simulink model "UAV_TAILSITTER_MODEL"  (R2023a)
settings: Solver=FixedStepAuto  StartTime=0.0  StopTime=60  FixedStep=0.001  RelTol=1e-3
libraries: vrlib x1
settings Model: Creator=kiqMC  LastModifiedBy=kiqMC
settings OptimizationCC: ReuseModelBlockBuffer=off

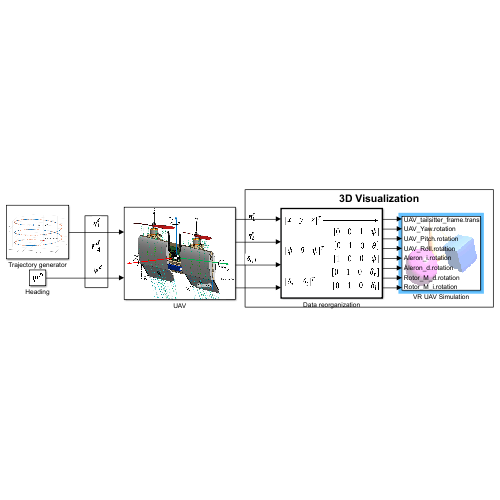
[thumbnail: Simulink's stored preview of the top-level diagram]
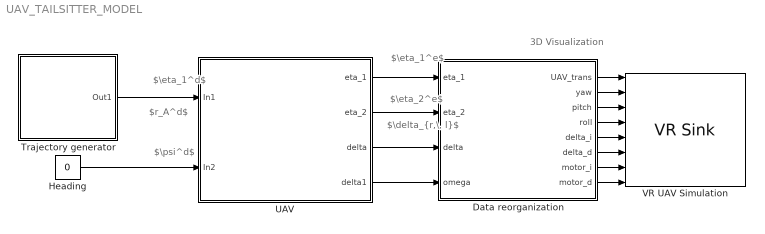
== system UAV_TAILSITTER_MODEL ==
  note: 3D Visualization
  note: $r_A^d$
  note: $\delta_{r,\, l}$
  note: $\eta_1^e$
  note: $\psi^d$
  note: $\eta_1^d$
  note: $\eta_2^e$
  Data reorganization : MATLAB Function  TreatAsAtomicUnit=on
  Heading : Constant  Value=0
      mask Display: image('C:\Users\kiqMC\Dropbox\Proyecto de Tesis MAC\psi_des.png'); % Use "Edit Image" on toolstrip to change.
  Trajectory generator : Subsystem
      mask Display: image('C:\Users\kiqMC\Dropbox\Proyecto de Tesis MAC\trajectoria.png'); % Use "Edit Image" on toolstrip to change.
  UAV : Subsystem
      mask Display: image('C:\Users\kiqMC\Dropbox\Tesis Enrique Mar\Modelo\Simulador UAV\Imágenes\UAV Fuerzas pares.png'); % Use "Edit Image" on toolstrip to change.
  VR UAV Simulation : vrlib/VR Sink  InstantiateOnLoad=on  SampleTime=0.05  ViewEnable=on  RemoteChange=off  RemoteView=off  FieldsWritten=UAV_tailsitter_frame.translation.3.1.1.double#UAV_Yaw.rotation.4.1.1.double#UAV_Pitch.rotation.4.1.1.double#UAV_Roll.rotation.4.1.1.double#Aleron_i.rotation.4.1.1.double#Aleron_d.rotation.4.1.1.double#Rotor_M_d.rotation.4.1.1.double#Rotor_M_i.rotation.4.1.1.double  WorldFileName=C:\Users\kiqMC\Dropbox\Proyecto de Tesis MAC\Diseño CAD drone\Tailsitter 0.3\UAV tailsitter ENSAMBLE MATLAB\uav world motors.wrl  AutoView=off  VideoDimensions=[]  AllowVariableSize=off
  wires:
  Trajectory generator/1(Out1) -> UAV/1(In1)
  UAV/1(eta_1) -> Data reorganization/1(eta_1)
  UAV/2(eta_2) -> Data reorganization/2(eta_2)
  UAV/3(delta) -> Data reorganization/3(delta)
  Heading/1 -> UAV/2(In2)
  UAV/4(delta1) -> Data reorganization/4(omega)
  Data reorganization/1(UAV_trans) -> VR UAV Simulation/1
  Data reorganization/2(yaw) -> VR UAV Simulation/2
  Data reorganization/3(pitch) -> VR UAV Simulation/3
  Data reorganization/4(roll) -> VR UAV Simulation/4
  Data reorganization/5(delta_i) -> VR UAV Simulation/5
  Data reorganization/6(delta_d) -> VR UAV Simulation/6
  Data reorganization/7(motor_i) -> VR UAV Simulation/7
  Data reorganization/8(motor_d) -> VR UAV Simulation/8

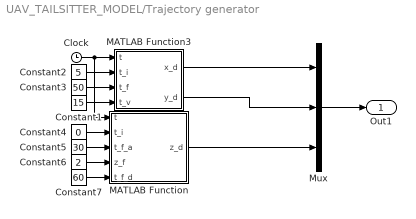
== system UAV_TAILSITTER_MODEL/Trajectory generator ==
  Clock : Clock
  Constant1 : Constant  Value=15
  Constant2 : Constant  Value=5
  Constant3 : Constant  Value=50
  Constant4 : Constant  Value=0
  Constant5 : Constant  Value=30
  Constant6 : Constant  Value=2
  Constant7 : Constant  Value=60
  MATLAB Function : MATLAB Function  TreatAsAtomicUnit=on
  MATLAB Function3 : MATLAB Function  TreatAsAtomicUnit=on
  Mux : Mux  Inputs=3
  Out1 : Outport
  wires:
  MATLAB Function/1(z_d) -> Mux/3
  Constant5/1 -> MATLAB Function/3(t_f_a)
  Constant7/1 -> MATLAB Function/5(t_f_d)
  Constant4/1 -> MATLAB Function/2(t_i)
  Clock/1 -> MATLAB Function/1(t), MATLAB Function3/1(t)
  Constant1/1 -> MATLAB Function3/4(t_v)
  MATLAB Function3/2(y_d) -> Mux/2
  Constant2/1 -> MATLAB Function3/2(t_i)
  MATLAB Function3/1(x_d) -> Mux/1
  Constant3/1 -> MATLAB Function3/3(t_f)
  Constant6/1 -> MATLAB Function/4(z_f)
  Mux/1 -> Out1/1

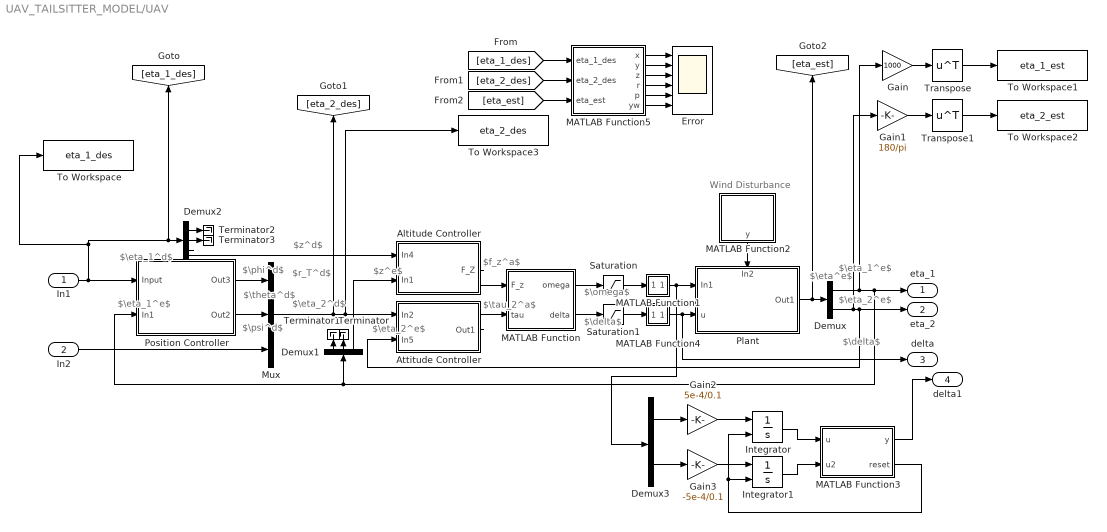
== system UAV_TAILSITTER_MODEL/UAV ==
  note: Wind Disturbance
  note: $\eta^e$
  note: $\eta_2^e$
  note: $\eta_1^e$
  note: $r_T^d$
  note: $z^d$
  note: $z^e$
  note: $\eta_1^d$
  note: $\eta_1^e$
  note: $\eta_2^d$
  note: $\tau_2^a$
  note: $\eta_2^e$
  note: $\omega$
  note: $f_z^a$
  note: $\delta$
  note: $\psi^d$
  note: $\phi^d$
  note: $\theta^d$
  note: $\delta$
  In1 : Inport
  In2 : Inport  Port=2
  Altitude Controller : Subsystem
      mask Display: image('C:\Users\kiqMC\Dropbox\Tesis Enrique Mar\Modelo\Simulador UAV\Imágenes\UAV altitud.png'); % Use "Edit Image" on toolstrip to change.
  Attitude Controller : Subsystem
      mask Display: image('C:\Users\kiqMC\Dropbox\Tesis Enrique Mar\Modelo\Simulador UAV\Imágenes\attitude.png'); % Use "Edit Image" on toolstrip to change.
  Demux : Demux  Outputs=2
  Demux1 : Demux  Outputs=3
  Demux2 : Demux  Outputs=3
  Demux3 : Demux  Outputs=2
  Error : Scope  NumInputPorts=6
  Gain : Gain  Gain=1000
  Gain1 : Gain  Gain=180/pi
  Gain2 : Gain  Gain=5e-4/0.1
  Gain3 : Gain  Gain=-5e-4/0.1
  Integrator : Integrator  ExternalReset=rising  InitialCondition=-180
  Integrator1 : Integrator  ExternalReset=rising  InitialCondition=180
  MATLAB Function : MATLAB Function  TreatAsAtomicUnit=on
  MATLAB Function1 : MATLAB Function  TreatAsAtomicUnit=on
  MATLAB Function2 : MATLAB Function  TreatAsAtomicUnit=on
  MATLAB Function3 : MATLAB Function  TreatAsAtomicUnit=on
  MATLAB Function4 : MATLAB Function  TreatAsAtomicUnit=on
  MATLAB Function5 : MATLAB Function  TreatAsAtomicUnit=on
  Mux : Mux  Inputs=3
  Plant : Subsystem
      settings: PortSchema="{\"entries\":[{\"content\":{\"sides\":[{\"content\":{\"connectorIds\":[\"In1\",\"In2\"]},\"type\":\"ConnectorPlacement.EquallySpacedRectSide\",\"uuid\":\"7724979e-19ed-4aea-9b0c-b20c5897cfe4\"},{\"content\":{\"connectorIds\":[\"Out1\"],\"side\":\"RIGHT\"},\"type\":\"ConnectorPlacement.EquallySpacedRectSide\",\"uuid\":\"79b46cc9-feaa-4989-867f-3ea67bf432a4\"},{\"content\":{\"connectorIds\":[\"In3\"],\"side\":\"TOP\"},\"type\":\"ConnectorPlacement.EquallySpacedRectSide\",\"uuid\":\"47fc0c27-c95e-4a7c-a970-96a958cf5736\"}]},\"type\":\"ConnectorPlacement.EquallySpacedConnector\",\"uuid\":\"a2521353-5775-4b64-ae3f-968c3914afab\"}],\"packageUris\":[\"http://schema.mathworks.com/mf0/Connector/R2020b\"],\"version\":\"1.0\"}"
      mask Display: image('C:\Users\kiqMC\Dropbox\Tesis Enrique Mar\Modelo\Simulador UAV\Imágenes\1.png'); % Use "Edit Image" on toolstrip to change.
  Position Controller : Subsystem
      mask Display: image('C:\Users\kiqMC\Dropbox\Tesis Enrique Mar\Modelo\Simulador UAV\Imágenes\position.png'); % Use "Edit Image" on toolstrip to change.
  Saturation : Saturate  UpperLimit=11000  LowerLimit=9600
  Saturation1 : Saturate  UpperLimit=10*pi/180  LowerLimit=-10*pi/180
  Terminator{,1..3} (4 alike) : Terminator
  To Workspace : ToWorkspace  VariableName=eta_1_des  SampleTime=-1
      settings: Save2DSignal=2-D array (concatenate along first dimension)
  To Workspace1 : ToWorkspace  VariableName=eta_1_est  SampleTime=-1
      settings: Save2DSignal=2-D array (concatenate along first dimension)
  To Workspace2 : ToWorkspace  VariableName=eta_2_est  SampleTime=-1
      settings: Save2DSignal=2-D array (concatenate along first dimension)
  To Workspace3 : ToWorkspace  VariableName=eta_2_des  SampleTime=-1
      settings: Save2DSignal=2-D array (concatenate along first dimension)
  Transpose : Math  Operator=transpose
  Transpose1 : Math  Operator=transpose
  eta_1 : Outport
  eta_2 : Outport  Port=2
  delta : Outport  Port=3
  delta1 : Outport  Port=4
  wires:
  [eta_1_des] -> MATLAB Function5/1(eta_1_des)
  Position Controller/1(Out3) -> Mux/1
  [eta_2_des] -> MATLAB Function5/2(eta_2_des)
  MATLAB Function5/5(p) -> Error/5
  MATLAB Function/1(omega) -> Saturation/1
  Demux2/3 -> Altitude Controller/1(In4)
  MATLAB Function1/1(y) -> Demux3/1, Plant/1(In1)
  Saturation/1 -> MATLAB Function1/1(u)
  Saturation1/1 -> MATLAB Function4/1(u)
  Demux/1 -> Gain/1, eta_1/1, Position Controller/2(In1), Demux1/1
  [eta_est] -> MATLAB Function5/3(eta_est)
  Plant/1(Out1) -> [eta_est], Demux/1
  MATLAB Function4/1(y) -> delta/1, Plant/2(u)
  Position Controller/2(Out2) -> Mux/2
  Demux/2 -> eta_2/1, Attitude Controller/2(In5), Gain1/1
  Demux2/2 -> Terminator3/1
  MATLAB Function5/3(z) -> Error/3
  Mux/1 -> [eta_2_des], To Workspace3/1, Attitude Controller/1(In2)
  Attitude Controller/1(Out1) -> MATLAB Function/2(tau)
  MATLAB Function5/4(r) -> Error/4
  Demux2/1 -> Terminator2/1
  Demux1/2 -> Terminator/1
  MATLAB Function/2(delta) -> Saturation1/1
  Demux1/1 -> Terminator1/1
  Demux1/3 -> Altitude Controller/2(In1)
  MATLAB Function5/2(y) -> Error/2
  MATLAB Function5/1(x) -> Error/1
  MATLAB Function5/6(yw) -> Error/6
  In1/1 -> Position Controller/1(Input), To Workspace/1, [eta_1_des], Demux2/1
  In2/1 -> Mux/3
  Altitude Controller/1(F_Z) -> MATLAB Function/1(F_z)
  MATLAB Function2/1(y) -> Plant/3(In2)
  Transpose/1 -> To Workspace1/1
  Transpose1/1 -> To Workspace2/1
  Gain/1 -> Transpose/1
  Gain1/1 -> Transpose1/1
  Integrator/1 -> MATLAB Function3/1(u)
  Gain2/1 -> Integrator/1
  MATLAB Function3/1(y) -> delta1/1
  MATLAB Function3/2(reset) -> Integrator/2, Integrator1/2
  Integrator1/1 -> MATLAB Function3/2(u2)
  Gain3/1 -> Integrator1/1
  Demux3/1 -> Gain2/1
  Demux3/2 -> Gain3/1

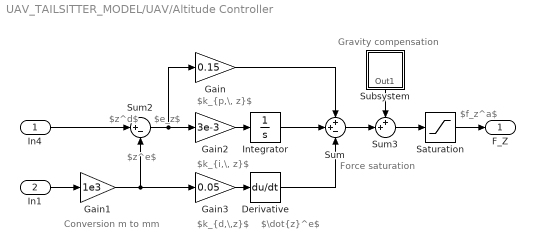
== system UAV_TAILSITTER_MODEL/UAV/Altitude Controller ==
  note: Conversion
      | m to mm
  note: $\dot{z}^e$
  note: $e_z$
  note: $f_z^a$
  note: Force saturation
  note: Gravity compensation
  note: $z^e$
  note: $z^d$
  note: $k_{p,\, z}$
  note: $k_{i,\, z}$
  note: $k_{d,\,z}$
  In4 : Inport
  In1 : Inport  Port=2
  Derivative : Derivative
  Gain : Gain  Gain=0.15
  Gain1 : Gain  Gain=1e3
  Gain2 : Gain  Gain=3e-3
  Gain3 : Gain  Gain=0.05
  Integrator : Integrator
  Saturation : Saturate  UpperLimit=13.791  LowerLimit=8.791
  Subsystem : Subsystem
      mask Display: image('C:\Users\kiqMC\Dropbox\Tesis Enrique Mar\Modelo\Simulador UAV\Imágenes\gravity.png'); % Use "Edit Image" on toolstrip to change.
  Sum : Sum  Inputs=++-
  Sum2 : Sum  Inputs=|+-
  Sum3 : Sum  Inputs=++|
  F_Z : Outport
  wires:
  Gain1/1 -> Sum2/2, Gain3/1
  In4/1 -> Sum2/1
  In1/1 -> Gain1/1
  Gain3/1 -> Derivative/1
  Gain2/1 -> Integrator/1
  Sum2/1 -> Gain2/1, Gain/1
  Integrator/1 -> Sum/2
  Gain/1 -> Sum/1
  Derivative/1 -> Sum/3
  Saturation/1 -> F_Z/1
  Sum/1 -> Sum3/2
  Sum3/1 -> Saturation/1
  Subsystem/1(Out1) -> Sum3/1

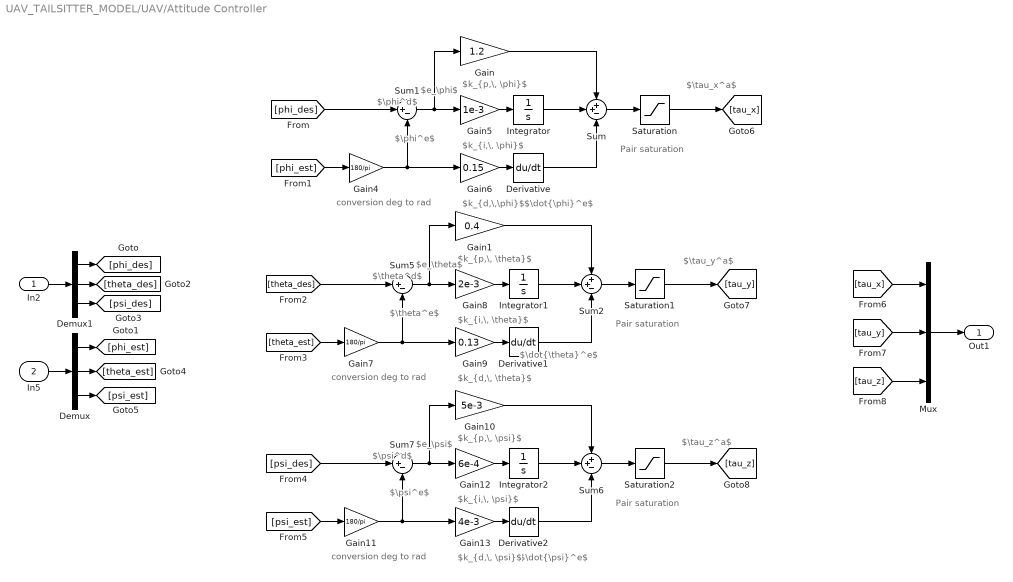
== system UAV_TAILSITTER_MODEL/UAV/Attitude Controller ==
  note: $\tau_z^a$
  note: $\tau_y^a$
  note: $\tau_x^a$
  note: conversion
      | deg to rad
  note: $e_\phi$
  note: $k_{i,\, \phi}$
  note: $\phi^d$
  note: $k_{d,\,\phi}$
  note: $\phi^e$
  note: $\dot{\phi}^e$
  note: $k_{p,\, \phi}$
  note: Pair saturation
  note: conversion
      | deg to rad
  note: $k_{d,\, \theta}$
  note: $k_{p,\, \theta}$
  note: $k_{i,\, \theta}$
  note: Pair saturation
  note: $\dot{\theta}^e$
  note: $\theta^e$
  note: $\theta^d$
  note: $e_\theta$
  note: $e_\psi$
  note: $\dot{\psi}^e$
  note: Pair saturation
  note: $\psi^d$
  note: $\psi^e$
  note: $k_{p,\, \psi}$
  note: $k_{i,\, \psi}$
  note: $k_{d,\, \psi}$
  note: conversion
      | deg to rad
  In2 : Inport
  In5 : Inport  Port=2
  Demux : Demux  Outputs=3
  Demux1 : Demux  Outputs=3
  Derivative : Derivative
  Derivative1 : Derivative
  Derivative2 : Derivative
  Gain : Gain  Gain=1.2
  Gain1 : Gain  Gain=0.4
  Gain10 : Gain  Gain=5e-3
  Gain11 : Gain  Gain=180/pi
  Gain12 : Gain  Gain=6e-4
  Gain13 : Gain  Gain=4e-3
  Gain4 : Gain  Gain=180/pi
  Gain5 : Gain  Gain=1e-3
  Gain6 : Gain  Gain=0.15
  Gain7 : Gain  Gain=180/pi
  Gain8 : Gain  Gain=2e-3
  Gain9 : Gain  Gain=0.13
  Integrator : Integrator
  Integrator1 : Integrator
  Integrator2 : Integrator
  Mux : Mux  Inputs=3
  Saturation : Saturate  UpperLimit=1.5  LowerLimit=-1.5
  Saturation1 : Saturate  UpperLimit=1.5  LowerLimit=-1.5
  Saturation2 : Saturate  UpperLimit=1.5  LowerLimit=-1.5
  Sum : Sum  Inputs=++-
  Sum1 : Sum  Inputs=|+-
  Sum2 : Sum  Inputs=++-
  Sum5 : Sum  Inputs=|+-
  Sum6 : Sum  Inputs=++-
  Sum7 : Sum  Inputs=|+-
  Out1 : Outport
  wires:
  In5/1 -> Demux/1
  Mux/1 -> Out1/1
  In2/1 -> Demux1/1
  Derivative/1 -> Sum/3
  Gain/1 -> Sum/1
  Gain4/1 -> Sum1/2, Gain6/1
  Gain5/1 -> Integrator/1
  Saturation/1 -> [tau_x]
  Gain6/1 -> Derivative/1
  Sum/1 -> Saturation/1
  Integrator/1 -> Sum/2
  Sum1/1 -> Gain5/1, Gain/1
  Demux1/1 -> [phi_des]
  Demux/1 -> [phi_est]
  [phi_des] -> Sum1/1
  [phi_est] -> Gain4/1
  Demux1/2 -> [theta_des]
  Demux1/3 -> [psi_des]
  Demux/2 -> [theta_est]
  Demux/3 -> [psi_est]
  [theta_des] -> Sum5/1
  [theta_est] -> Gain7/1
  Sum5/1 -> Gain8/1, Gain1/1
  Integrator1/1 -> Sum2/2
  Gain7/1 -> Sum5/2, Gain9/1
  Gain9/1 -> Derivative1/1
  Gain8/1 -> Integrator1/1
  Derivative1/1 -> Sum2/3
  Gain1/1 -> Sum2/1
  Sum2/1 -> Saturation1/1
  Saturation1/1 -> [tau_y]
  Gain13/1 -> Derivative2/1
  Sum7/1 -> Gain12/1, Gain10/1
  Integrator2/1 -> Sum6/2
  [psi_est] -> Gain11/1
  Derivative2/1 -> Sum6/3
  Gain12/1 -> Integrator2/1
  Gain10/1 -> Sum6/1
  Gain11/1 -> Sum7/2, Gain13/1
  Sum6/1 -> Saturation2/1
  [psi_des] -> Sum7/1
  Saturation2/1 -> [tau_z]
  [tau_x] -> Mux/1
  [tau_y] -> Mux/2
  [tau_z] -> Mux/3

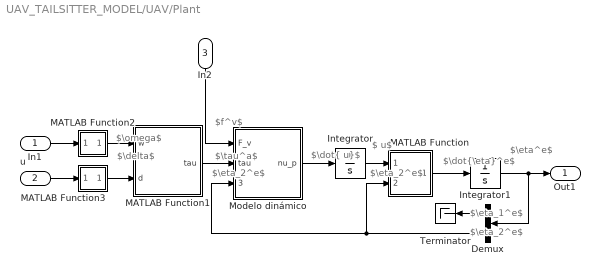
== system UAV_TAILSITTER_MODEL/UAV/Plant ==
  note: $f^v$
  note: $\tau^a$
  note: $\delta$
  note: $\omega$
  note: $\eta_1^e$
  note: $\dot{\eta}^e$
  note: $\eta^e$
  note: $\eta_2^e$
  note: $\nu$
  note: $\eta_2^e$
  note: $\dot{\nu}$
  note: $\eta_2^e$
  In1 : Inport
  u : Inport  Port=2
  In2 : Inport  Port=3
  Demux : Demux  Outputs=2
  Integrator : Integrator  InitialCondition=[0;0;0;0;0;0]
  Integrator1 : Integrator  InitialCondition=[0;0;0;0;0;0]  LowerSaturationLimit=[-inf;-inf;0;-inf; -inf;-inf]
  MATLAB Function : MATLAB Function  TreatAsAtomicUnit=on
  MATLAB Function1 : MATLAB Function  TreatAsAtomicUnit=on
  MATLAB Function2 : MATLAB Function  TreatAsAtomicUnit=on
  MATLAB Function3 : MATLAB Function  TreatAsAtomicUnit=on
  Modelo dinámico : MATLAB Function  TreatAsAtomicUnit=on
  Terminator : Terminator
  Out1 : Outport
  wires:
  MATLAB Function/1(q_d_r) -> Integrator1/1
  Integrator/1 -> MATLAB Function/1(q_d)
  Modelo dinámico/1(nu_p) -> Integrator/1
  Integrator1/1 -> Out1/1, Demux/1
  Demux/2 -> MATLAB Function/2(attitude), Modelo dinámico/3(attitude)
  Demux/1 -> Terminator/1
  MATLAB Function1/1(tau) -> Modelo dinámico/2(tau)
  In1/1 -> MATLAB Function2/1(u)
  MATLAB Function2/1(y) -> MATLAB Function1/1(w)
  u/1 -> MATLAB Function3/1(u)
  MATLAB Function3/1(y) -> MATLAB Function1/2(d)
  In2/1 -> Modelo dinámico/1(F_v)

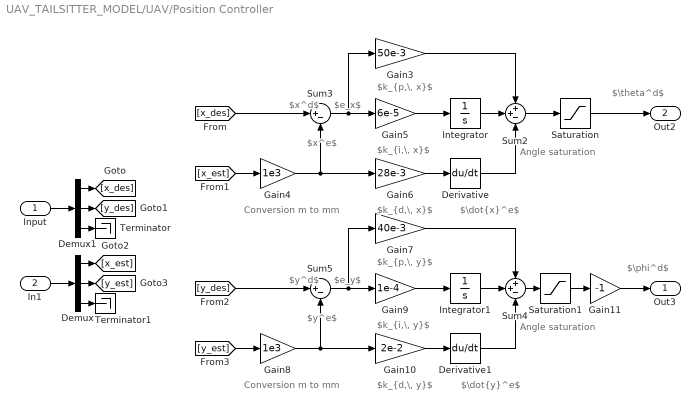
== system UAV_TAILSITTER_MODEL/UAV/Position Controller ==
  note: $e_x$
  note: $k_{i,\, x}$
  note: $x^d$
  note: $k_{d,\, x}$
  note: $x^e$
  note: $\dot{x}^e$
  note: $k_{p,\, x}$
  note: $\theta^d$
  note: Angle saturation
  note: Conversion
      | m to mm
  note: $e_y$
  note: $y^e$
  note: $y^d$
  note: $k_{i,\, y}$
  note: $\dot{y}^e$
  note: Angle saturation
  note: $k_{d,\, y}$
  note: $\phi^d$
  note: Conversion
      | m to mm
  note: $k_{p,\, y}$
  Input : Inport
  In1 : Inport  Port=2
  Demux : Demux  Outputs=3
  Demux1 : Demux  Outputs=3
  Derivative : Derivative
  Derivative1 : Derivative
  Gain10 : Gain  Gain=2e-2
  Gain11 : Gain  Gain=-1
  Gain3 : Gain  Gain=50e-3
  Gain4 : Gain  Gain=1e3
  Gain5 : Gain  Gain=6e-5
  Gain6 : Gain  Gain=28e-3
  Gain7 : Gain  Gain=40e-3
  Gain8 : Gain  Gain=1e3
  Gain9 : Gain  Gain=1e-4
  Integrator : Integrator
  Integrator1 : Integrator
  Saturation : Saturate  UpperLimit=10  LowerLimit=-10
  Saturation1 : Saturate  UpperLimit=10  LowerLimit=-10
  Sum2 : Sum  Inputs=++-
  Sum3 : Sum  Inputs=|+-
  Sum4 : Sum  Inputs=++-
  Sum5 : Sum  Inputs=|+-
  Terminator : Terminator
  Terminator1 : Terminator
  Out3 : Outport
  Out2 : Outport  Port=2
  wires:
  In1/1 -> Demux/1
  Input/1 -> Demux1/1
  Demux1/3 -> Terminator/1
  Demux/3 -> Terminator1/1
  Derivative/1 -> Sum2/3
  Gain3/1 -> Sum2/1
  Gain4/1 -> Sum3/2, Gain6/1
  [x_des] -> Sum3/1
  Gain5/1 -> Integrator/1
  Gain6/1 -> Derivative/1
  Sum2/1 -> Saturation/1
  Integrator/1 -> Sum2/2
  Sum3/1 -> Gain5/1, Gain3/1
  [x_est] -> Gain4/1
  Demux1/1 -> [x_des]
  Demux1/2 -> [y_des]
  Demux/1 -> [x_est]
  Saturation/1 -> Out2/1
  [y_des] -> Sum5/1
  Integrator1/1 -> Sum4/2
  Gain7/1 -> Sum4/1
  Gain8/1 -> Sum5/2, Gain10/1
  Sum4/1 -> Saturation1/1
  Sum5/1 -> Gain9/1, Gain7/1
  Derivative1/1 -> Sum4/3
  [y_est] -> Gain8/1
  Gain10/1 -> Derivative1/1
  Gain9/1 -> Integrator1/1
  Demux/2 -> [y_est]
  Saturation1/1 -> Gain11/1
  Gain11/1 -> Out3/1

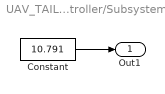
== system UAV_TAILSITTER_MODEL/UAV/Altitude Controller/Subsystem ==
  Constant : Constant  Value=10.791
  Out1 : Outport
  wires:
  Constant/1 -> Out1/1

== matlab function UAV_TAILSITTER_MODEL/UAV/Plant/MATLAB Function2 ==
  data: u input; y output
function y = fcn(u)

y = u;

== matlab function UAV_TAILSITTER_MODEL/UAV/Plant/MATLAB Function3 ==
  data: u input; y output
function y = fcn(u)

y = u;

== matlab function UAV_TAILSITTER_MODEL/Trajectory generator/MATLAB Function ==
  data: t input; t_i input; t_f_a input; z_f input; t_f_d input; z_d output
function z_d = fcn(t,t_i, t_f_a, z_f, t_f_d)

z_d = 0;
z_i = 0;
if t >= t_i && t < t_f_a
    z_d = ((z_i - z_f)/(t_i-t_f_a))*t;
else
    z_d = z_f + ((z_f - z_i)/(t_f_a-t_f_d))*(t-t_f_a);
end

z_d = z_d * 1000;

== matlab function UAV_TAILSITTER_MODEL/UAV/MATLAB Function2 ==
  data: y output
function y = fcn()

y = 0;

== matlab function UAV_TAILSITTER_MODEL/UAV/MATLAB Function3 ==
  data: u input; y output; reset output; u2 input
function [y, reset] = fcn(u, u2)
if u>180
    reset = 1;
else
    reset = 0;
end

y = [u; u2];

== matlab function UAV_TAILSITTER_MODEL/UAV/MATLAB Function1 ==
  data: u input; y output
function y = fcn(u)
y=u;
%y = (u-900)*13.0833333;

== matlab function UAV_TAILSITTER_MODEL/UAV/Plant/Modelo dinámico ==
  data: F_v input; tau input; nu_p output; attitude input
function nu_p = fcn(F_v, tau, attitude)

nu_p    = zeros(6,1);
F_g     =  zeros(3,1);
phi     = attitude(1);
theta   = attitude(2);
psi     = attitude(3);

F_a = tau(1:3);
tau_a = tau(4:6);

%% Definición de parámetros

m = 1.1;
g = -9.81;
%g = 0;

%% Matriz de rotación 
R_inv = [                             cos(psi)*cos(theta),                              cos(theta)*sin(psi),         -sin(theta);...
         cos(psi)*sin(phi)*sin(theta) - cos(phi)*sin(psi), cos(phi)*cos(psi) + sin(phi)*sin(psi)*sin(theta), cos(theta)*sin(phi);...
         sin(phi)*sin(psi) + cos(phi)*cos(psi)*sin(theta), cos(phi)*sin(psi)*sin(theta) - cos(psi)*sin(phi), cos(phi)*cos(theta)];

%% Rotación del vector de gravedad y cálculo de F_g

F_g = R_inv*[0;0;m*g];


%% Matriz de ceros
ceros_3_x_3 = [0    0   0;...
               0    0   0;...
               0    0   0];
%% Matriz de masas ivn
m_I_3_x_3 =   [1/m    0   0;  
               0    1/m   0;  
               0    0   1/m];
%% Matriz de inercias inv
J = [1/0.03269        0       0;...
           0     1/0.0056     0;...
           0        0    1/0.02712];
%% Matriz de masas e inercias inversa
M_inv = [m_I_3_x_3      ceros_3_x_3;...
         ceros_3_x_3        J];
%% Vector nu_p de aceleraciones lineales y angulares
tau_cm = zeros(3,1);
nu_p =  M_inv*[F_a  +   F_g +   F_v;...
               tau_a  + tau_cm    ];

== matlab function UAV_TAILSITTER_MODEL/UAV/Plant/MATLAB Function ==
  data: q_d input; attitude input size=3; q_d_r output
function q_d_r   = fcn(q_d, attitude)
phi = attitude(1);
theta = attitude(2);
psi = attitude(3);
%% Cálculo de la matriz de rotación 
% R_1 = [ cos(phi)*cos(theta), cos(psi)*sin(phi) + cos(phi)*sin(psi)*sin(theta), sin(phi)*sin(psi) - cos(phi)*cos(psi)*sin(theta);...
%          -cos(theta)*sin(phi), cos(phi)*cos(psi) - sin(phi)*sin(psi)*sin(theta), cos(phi)*sin(psi) + cos(psi)*sin(phi)*sin(theta);...
%           sin(theta),                             -cos(theta)*sin(psi),                              cos(psi)*cos(theta)];

R_1 = [ cos(psi)*cos(theta), cos(psi)*sin(phi)*sin(theta) - cos(phi)*sin(psi), sin(phi)*sin(psi) + cos(phi)*cos(psi)*sin(theta);...
        cos(theta)*sin(psi), cos(phi)*cos(psi) + sin(phi)*sin(psi)*sin(theta), cos(phi)*sin(psi)*sin(theta) - cos(psi)*sin(phi);...
                -sin(theta),                              cos(theta)*sin(phi),                              cos(phi)*cos(theta)];

%% Rotación del vector de velocidades lineales xi_d
xi_d_rot = R_1*[q_d(1);   q_d(2);     q_d(3)];

%% Cálculo de la matriz de rotación para la velocidades angulares
R_2 = [1    sin(phi)*tan(theta)     cos(phi)*tan(theta);...
       0        cos(phi)                      -sin(phi);...
       0    sin(phi)/cos(theta)     cos(phi)/cos(theta)];

%% Rotación del vector de velocidades angulares eta_d
eta_d_rot = R_2*[q_d(4);  q_d(5);     q_d(6)];

%% Formación del vector de velocidades lineales y angulares q_d_rot
q_d_r = [xi_d_rot;    eta_d_rot];

== matlab function UAV_TAILSITTER_MODEL/UAV/MATLAB Function ==
  data: F_z input; omega output; tau input; delta output
function [omega, delta] = fcn(F_z, tau)

G_r = 5.0143209e-8;
G_l = 5.0143209e-8;
a = 195.07841077/1000;
b = 91.34348944/1000;

F_a_z = F_z;
tau_a_x = tau(1);
tau_a_y = tau(2);
tau_a_z = tau(3);

omega = [sqrt((a*F_a_z + tau_a_x)/(2*a*G_r));
         sqrt((a*F_a_z - tau_a_x)/(2*a*G_l))];

delta = [(-b*tau_a_z - a*tau_a_y)/(b*(a*F_a_z + tau_a_x));
         ( b*tau_a_z - a*tau_a_y)/(b*(a*F_a_z - tau_a_x))];

== matlab function UAV_TAILSITTER_MODEL/UAV/Plant/MATLAB Function1 ==
  data: w input; tau output; d input
function tau = fcn(w, d)
    r = 1; l = 2; % 
    tau = zeros(6,1);
    Gp = [5.0143209e-8; 5.0143209e-8]; % Ganancias de propulsión 
    a   = 0.1950784; % Distancia del brazo de palanca "a" al c.m.
    b   = 0.0913434; % Distancia del brazo de palanca "b" al c.m.
    
    % Fuerzas de actuación, omeGpa -> w y delta -> d
    F_a =[ -(Gp(r)*w(r)^2*d(r)  +   Gp(l)*w(l)^2*d(l));...
                                0                     ;...
             Gp(r)*w(r)^2       +   Gp(l)*w(l)^2];
    
    % Pares de actuación 
    tau_a = [ a*(Gp(r)*w(r)^2        -  Gp(l)*w(l)^2);...
             -b*(Gp(r)*w(r)^2*d(r)   +  Gp(l)*w(l)^2*d(l));...
             -a*(Gp(r)*w(r)^2*d(r)   -  Gp(l)*w(l)^2*d(l))];
    
    % Vector de fuerzas y pares de actuación
    tau = [F_a; tau_a];

== matlab function UAV_TAILSITTER_MODEL/UAV/MATLAB Function4 ==
  data: u input; y output
function y = fcn(u)

y = u;

%7333.37

== matlab function UAV_TAILSITTER_MODEL/Data reorganization ==
  data: eta_1 input; UAV_trans output; eta_2 input; yaw output; pitch output; roll output; delta input; delta_i output; delta_d output; omega input; motor_i output; motor_d output
function [UAV_trans ,yaw, pitch, roll, delta_i, delta_d,motor_i, motor_d] = fcn(eta_1 ,eta_2, delta, omega)

    roll    = [1; 0; 0; eta_2(1)];
    pitch   = [0; 1; 0; eta_2(2)];
    yaw     = [0; 0; 1; eta_2(3)];
    
    delta_i = [0; 1; 0; delta(1)];
    delta_d = [0; 1; 0; delta(2)];
    motor_i = [0; 0; 1; omega(1)];
    motor_d = [0; 0; 1; omega(2)];
    
    UAV_trans = eta_1*1000;

== matlab function UAV_TAILSITTER_MODEL/Trajectory generator/MATLAB Function3 ==
  data: t input; x_d output; t_i input; t_f input; t_v input; y_d output
function [x_d, y_d] = fcn(t, t_i, t_f, t_v)
x_d = 0;
y_d = 0;
radi = 1000;

if t_i < t && t < t_f
    x_d = radi*cos(2*pi*((t-t_i)/t_v))-radi;
    y_d = radi*sin(2*pi*((t-t_i)/t_v));
end

== matlab function UAV_TAILSITTER_MODEL/UAV/MATLAB Function5 ==
  data: x output; eta_1_des input; y output; eta_2_des input; eta_est input; z output; r output; p output; yw output
function [x, y, z, r, p, yw] = fcn(eta_1_des, eta_2_des, eta_est)

x = [eta_1_des(1)/1000; eta_est(1)];
y = [eta_1_des(2)/1000; eta_est(2)];
z = [eta_1_des(3)/1000; eta_est(3)];
r = [eta_2_des(1)*pi/180; eta_est(4)];
p = [eta_2_des(2)*pi/180; eta_est(5)];
yw = [eta_2_des(3)*pi/180; eta_est(6)];
